simulink model "run_2022"  (R2022b)
settings: Solver=VariableStepAuto  StartTime=t_i  StopTime=2  MaxStep=s_max  RelTol=1e-3
InitFcn:
  | data;
  | init;
values from neighbouring files (symbols this model uses):
  h_ej = 0.15    [data.m]
  phi_0 = atan(-(r_ej*h_0)/(h_ej^2*sqrt(1-h_0^2/h_ej^2)))    [init.m]
  r_0 = sqrt((r_ej^2)*(1-h_0^2/h_ej^2))    [init.m]
  r_ej = 0.0821    [data.m]
  T_d = 1e-20    [data.m]
  x_ej = -0.05    [data.m]
  y_ej = 0.06    [data.m]
  z_ej = -0.03    [data.m]
undefined symbols (not defined in the file or in its folder): Glenohumeral_F0M, Glenohumeral_l0, Scapulothoracic_F0M, Scapulothoracic_l0, X, Y, Z
libraries: sm_lib x148, nesl_utility x62
(part 2 of 4)

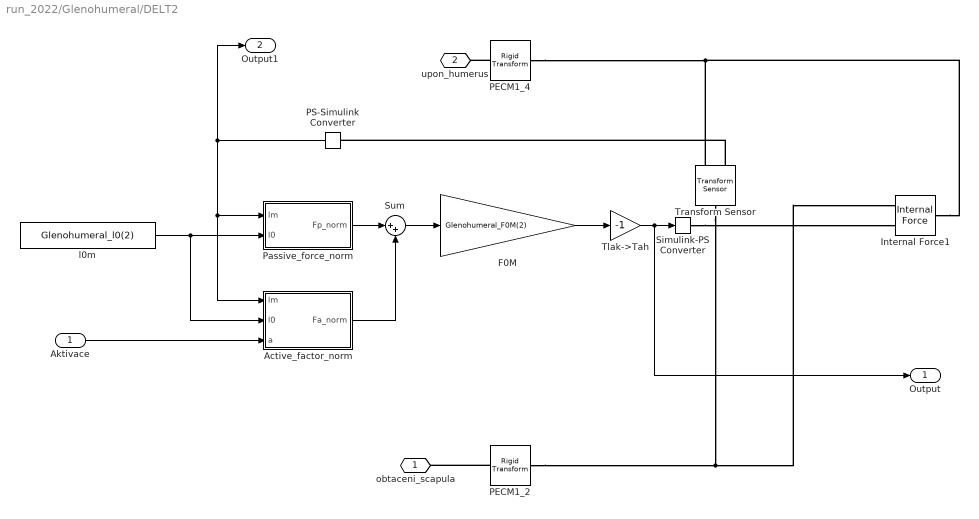
== system run_2022/Glenohumeral/DELT2 ==
  Aktivace : Inport
  Active_factor_norm : MATLAB Function  TreatAsAtomicUnit=on
  F0M : Gain  Gain=Glenohumeral_F0M(2)
  Internal Force1 : sm_lib/Forces and Torques/Internal Force
  PECM1_2 : sm_lib/Frames and Transforms/Rigid Transform  TranslationMethod=Cartesian  TranslationStandardOffset=0  TranslationStandardOffsetUnits=m  TranslationStandardAxis=+Z  TranslationCartesianOffset=[-0.028 -0.005 0.018]  TranslationCartesianOffsetUnits=m  TranslationROffset=0  TranslationROffsetUnits=m  TranslationZOffset=0  TranslationZOffsetUnits=m  TranslationThetaOffset=0  TranslationThetaOffsetUnits=deg  RotationMethod=None  RotationAngleUnits=deg  RotationStandardAxis=+Z  RotationAngle=0.0  RotationArbitraryAxis=[0 0 1]  FollAlignAxisA=+X  BaseAlignAxisA=+Y  FollAlignAxisB=+Y  BaseAlignAxisB=+Z  RotationSequenceAxes=FollowerAxes  RotationSequence=XYX  RotationSequenceAngles=[0 0 0]  RotationSequenceAnglesUnits=deg  RotationMatrix=[1 0 0; 0 1 0; 0 0 1]  Quaternion=[1 0 0 0]
  PECM1_4 : sm_lib/Frames and Transforms/Rigid Transform  TranslationMethod=Cartesian  TranslationStandardOffset=0  TranslationStandardOffsetUnits=m  TranslationStandardAxis=+Z  TranslationCartesianOffset=[-0.004 -0.058 0.028]  TranslationCartesianOffsetUnits=m  TranslationROffset=0  TranslationROffsetUnits=m  TranslationZOffset=0  TranslationZOffsetUnits=m  TranslationThetaOffset=0  TranslationThetaOffsetUnits=deg  RotationMethod=StandardAxis  RotationAngleUnits=deg  RotationStandardAxis=+Y  RotationAngle=90  RotationArbitraryAxis=[0 0 1]  FollAlignAxisA=+X  BaseAlignAxisA=+Y  FollAlignAxisB=+Y  BaseAlignAxisB=+Z  RotationSequenceAxes=FollowerAxes  RotationSequence=XYX  RotationSequenceAngles=[0 0 0]  RotationSequenceAnglesUnits=deg  RotationMatrix=[1 0 0; 0 1 0; 0 0 1]  Quaternion=[1 0 0 0]
  PS-Simulink Converter : nesl_utility/PS-Simulink Converter  PhysicalDomain=network_engine_domain  SubClassName=ps_output  LeftPortType=input  RightPortType=output  PseudoPeriodic=off  Frequencies=[]  VectorFormat=inherit  Unit=inherit  AffineConversion=off
  Passive_force_norm : MATLAB Function  TreatAsAtomicUnit=on
  Simulink-PS Converter : nesl_utility/Simulink-PS Converter  PhysicalDomain=network_engine_domain  SubClassName=ps_input  LeftPortType=input  RightPortType=output  PseudoPeriodic=off  Frequencies=[]  NoiseDistribution=none  NoiseParameters=[]  Unit=1  AffineConversion=off  FilteringAndDerivatives=provide  SimscapeFilterOrder=1  InputFilterTimeConstant=0.001  UdotUserProvided=0
  Sum : Sum  Inputs=|++
  Tlak->Tah : Gain  Gain=-1
  Transform Sensor : sm_lib/Frames and Transforms/Transform Sensor  MeasurementFrame=World  RotationSequence=XYX  SenseAngle=off  SenseAxis=off  SenseQ=off  SenseR=off  SenseRotationSequence=off  SenseOmegaX=off  SenseOmegaY=off  SenseOmegaZ=off  SenseQDot=off  SenseRDot=off  SenseRotationSequenceDot=off  SenseAlphaX=off  SenseAlphaY=off  SenseAlphaZ=off  SenseQDDot=off  SenseRDDot=off  SenseX=off  SenseY=off  SenseZ=off  SenseRad=off  SenseAzim=off  SenseDist=on  SenseInc=off  SenseXDot=off  SenseYDot=off  SenseZDot=off  SenseRadDot=off  SenseAzimDot=off  SenseDistDot=off  SenseIncDot=off  SenseXDDot=off  SenseYDDot=off  SenseZDDot=off  SenseRadDDot=off  SenseAzimDDot=off  SenseDistDDot=off  SenseIncDDot=off
  l0m : Constant  Value=Glenohumeral_l0(2)
  obtaceni_scapula : PMIOPort  Side=Left
  upon_humerus : PMIOPort  Port=2  Side=Left
  Output : Outport
  Output1 : Outport  Port=2
  wires:
  Passive_force_norm/1(Fp_norm) -> Sum/1
  F0M/1 -> Tlak->Tah/1
  Sum/1 -> F0M/1
  Active_factor_norm/1(Fa_norm) -> Sum/2
  Tlak->Tah/1 -> Output/1, Simulink-PS Converter/1
  PS-Simulink Converter/1 -> Output1/1, Active_factor_norm/1(lm), Passive_force_norm/1(lm)
  l0m/1 -> Active_factor_norm/2(l0), Passive_force_norm/2(l0)
  Aktivace/1 -> Active_factor_norm/3(a)
  connections:
  Transform Sensor/LConn1 -- PECM1_2/RConn1 -- Internal Force1/LConn1
  Transform Sensor/RConn1 -- PECM1_4/RConn1 -- Internal Force1/RConn1
  PECM1_2/LConn1 -- obtaceni_scapula/RConn1
  PECM1_4/LConn1 -- upon_humerus/RConn1
  Simulink-PS Converter/RConn1 -- Internal Force1/LConn2
  Transform Sensor/RConn2 -- PS-Simulink Converter/LConn1

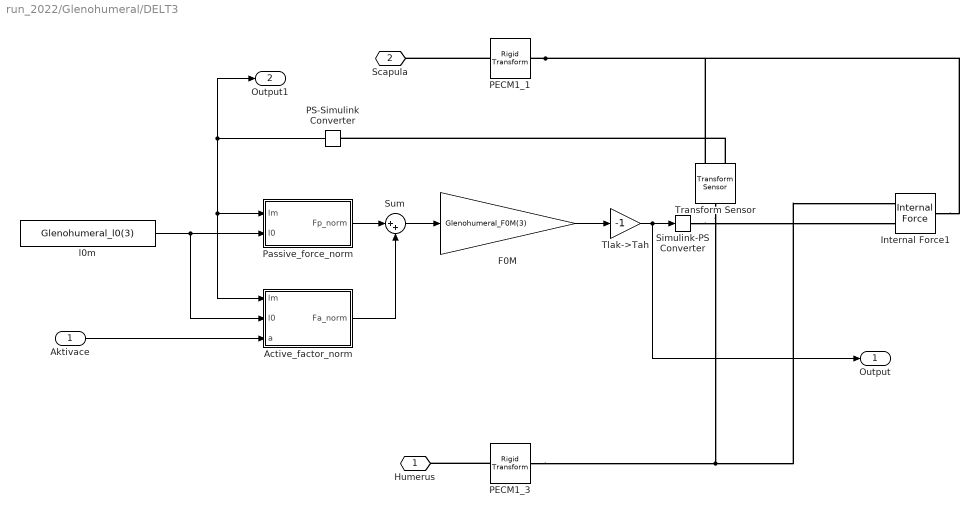
== system run_2022/Glenohumeral/DELT3 ==
  Aktivace : Inport
  Active_factor_norm : MATLAB Function  TreatAsAtomicUnit=on
  F0M : Gain  Gain=Glenohumeral_F0M(3)
  Internal Force1 : sm_lib/Forces and Torques/Internal Force
  PECM1_1 : sm_lib/Frames and Transforms/Rigid Transform  TranslationMethod=Cartesian  TranslationStandardOffset=0  TranslationStandardOffsetUnits=m  TranslationStandardAxis=+Z  TranslationCartesianOffset=[-0.072 -0.024 0.006]  TranslationCartesianOffsetUnits=m  TranslationROffset=0  TranslationROffsetUnits=m  TranslationZOffset=0  TranslationZOffsetUnits=m  TranslationThetaOffset=0  TranslationThetaOffsetUnits=deg  RotationMethod=None  RotationAngleUnits=deg  RotationStandardAxis=+Z  RotationAngle=0.0  RotationArbitraryAxis=[0 0 1]  FollAlignAxisA=+X  BaseAlignAxisA=+Y  FollAlignAxisB=+Y  BaseAlignAxisB=+Z  RotationSequenceAxes=FollowerAxes  RotationSequence=XYX  RotationSequenceAngles=[0 0 0]  RotationSequenceAnglesUnits=deg  RotationMatrix=[1 0 0; 0 1 0; 0 0 1]  Quaternion=[1 0 0 0]
  PECM1_3 : sm_lib/Frames and Transforms/Rigid Transform  TranslationMethod=Cartesian  TranslationStandardOffset=0  TranslationStandardOffsetUnits=m  TranslationStandardAxis=+Z  TranslationCartesianOffset=[-0.019 -0.05 0.006]  TranslationCartesianOffsetUnits=m  TranslationROffset=0  TranslationROffsetUnits=m  TranslationZOffset=0  TranslationZOffsetUnits=m  TranslationThetaOffset=0  TranslationThetaOffsetUnits=deg  RotationMethod=StandardAxis  RotationAngleUnits=deg  RotationStandardAxis=+Y  RotationAngle=90  RotationArbitraryAxis=[0 0 1]  FollAlignAxisA=+X  BaseAlignAxisA=+Y  FollAlignAxisB=+Y  BaseAlignAxisB=+Z  RotationSequenceAxes=FollowerAxes  RotationSequence=XYX  RotationSequenceAngles=[0 0 0]  RotationSequenceAnglesUnits=deg  RotationMatrix=[1 0 0; 0 1 0; 0 0 1]  Quaternion=[1 0 0 0]
  PS-Simulink Converter : nesl_utility/PS-Simulink Converter  PhysicalDomain=network_engine_domain  SubClassName=ps_output  LeftPortType=input  RightPortType=output  PseudoPeriodic=off  Frequencies=[]  VectorFormat=inherit  Unit=inherit  AffineConversion=off
  Passive_force_norm : MATLAB Function  TreatAsAtomicUnit=on
  Simulink-PS Converter : nesl_utility/Simulink-PS Converter  PhysicalDomain=network_engine_domain  SubClassName=ps_input  LeftPortType=input  RightPortType=output  PseudoPeriodic=off  Frequencies=[]  NoiseDistribution=none  NoiseParameters=[]  Unit=1  AffineConversion=off  FilteringAndDerivatives=provide  SimscapeFilterOrder=1  InputFilterTimeConstant=0.001  UdotUserProvided=0
  Sum : Sum  Inputs=|++
  Tlak->Tah : Gain  Gain=-1
  Transform Sensor : sm_lib/Frames and Transforms/Transform Sensor  MeasurementFrame=World  RotationSequence=XYX  SenseAngle=off  SenseAxis=off  SenseQ=off  SenseR=off  SenseRotationSequence=off  SenseOmegaX=off  SenseOmegaY=off  SenseOmegaZ=off  SenseQDot=off  SenseRDot=off  SenseRotationSequenceDot=off  SenseAlphaX=off  SenseAlphaY=off  SenseAlphaZ=off  SenseQDDot=off  SenseRDDot=off  SenseX=off  SenseY=off  SenseZ=off  SenseRad=off  SenseAzim=off  SenseDist=on  SenseInc=off  SenseXDot=off  SenseYDot=off  SenseZDot=off  SenseRadDot=off  SenseAzimDot=off  SenseDistDot=off  SenseIncDot=off  SenseXDDot=off  SenseYDDot=off  SenseZDDot=off  SenseRadDDot=off  SenseAzimDDot=off  SenseDistDDot=off  SenseIncDDot=off
  l0m : Constant  Value=Glenohumeral_l0(3)
  Humerus : PMIOPort  Side=Left
  Scapula : PMIOPort  Port=2  Side=Left
  Output : Outport
  Output1 : Outport  Port=2
  wires:
  l0m/1 -> Active_factor_norm/2(l0), Passive_force_norm/2(l0)
  Tlak->Tah/1 -> Output/1, Simulink-PS Converter/1
  PS-Simulink Converter/1 -> Output1/1, Active_factor_norm/1(lm), Passive_force_norm/1(lm)
  Active_factor_norm/1(Fa_norm) -> Sum/2
  Sum/1 -> F0M/1
  Passive_force_norm/1(Fp_norm) -> Sum/1
  F0M/1 -> Tlak->Tah/1
  Aktivace/1 -> Active_factor_norm/3(a)
  connections:
  PECM1_1/RConn1 -- Internal Force1/RConn1 -- Transform Sensor/RConn1
  PECM1_3/RConn1 -- Internal Force1/LConn1 -- Transform Sensor/LConn1
  Transform Sensor/RConn2 -- PS-Simulink Converter/LConn1
  Simulink-PS Converter/RConn1 -- Internal Force1/LConn2
  PECM1_3/LConn1 -- Humerus/RConn1
  PECM1_1/LConn1 -- Scapula/RConn1

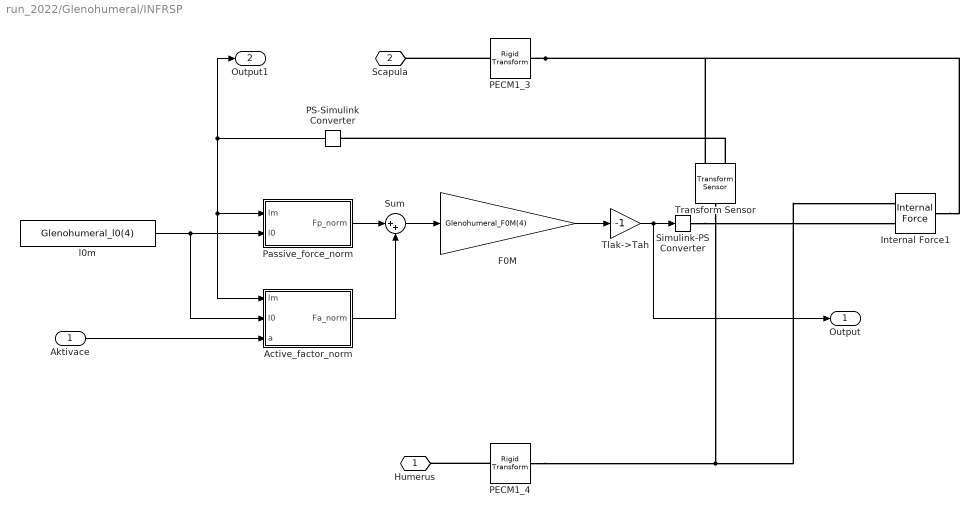
== system run_2022/Glenohumeral/INFRSP ==
  Aktivace : Inport
  Active_factor_norm : MATLAB Function  TreatAsAtomicUnit=on
  F0M : Gain  Gain=Glenohumeral_F0M(4)
  Internal Force1 : sm_lib/Forces and Torques/Internal Force
  PECM1_3 : sm_lib/Frames and Transforms/Rigid Transform  TranslationMethod=Cartesian  TranslationStandardOffset=0  TranslationStandardOffsetUnits=m  TranslationStandardAxis=+Z  TranslationCartesianOffset=[-0.043 -0.048 -0.022]  TranslationCartesianOffsetUnits=m  TranslationROffset=0  TranslationROffsetUnits=m  TranslationZOffset=0  TranslationZOffsetUnits=m  TranslationThetaOffset=0  TranslationThetaOffsetUnits=deg  RotationMethod=None  RotationAngleUnits=deg  RotationStandardAxis=+Z  RotationAngle=0.0  RotationArbitraryAxis=[0 0 1]  FollAlignAxisA=+X  BaseAlignAxisA=+Y  FollAlignAxisB=+Y  BaseAlignAxisB=+Z  RotationSequenceAxes=FollowerAxes  RotationSequence=XYX  RotationSequenceAngles=[0 0 0]  RotationSequenceAnglesUnits=deg  RotationMatrix=[1 0 0; 0 1 0; 0 0 1]  Quaternion=[1 0 0 0]
  PECM1_4 : sm_lib/Frames and Transforms/Rigid Transform  TranslationMethod=Cartesian  TranslationStandardOffset=0  TranslationStandardOffsetUnits=m  TranslationStandardAxis=+Z  TranslationCartesianOffset=[-0.005 0.008 0.026]  TranslationCartesianOffsetUnits=m  TranslationROffset=0  TranslationROffsetUnits=m  TranslationZOffset=0  TranslationZOffsetUnits=m  TranslationThetaOffset=0  TranslationThetaOffsetUnits=deg  RotationMethod=StandardAxis  RotationAngleUnits=deg  RotationStandardAxis=+Y  RotationAngle=90  RotationArbitraryAxis=[0 0 1]  FollAlignAxisA=+X  BaseAlignAxisA=+Y  FollAlignAxisB=+Y  BaseAlignAxisB=+Z  RotationSequenceAxes=FollowerAxes  RotationSequence=XYX  RotationSequenceAngles=[0 0 0]  RotationSequenceAnglesUnits=deg  RotationMatrix=[1 0 0; 0 1 0; 0 0 1]  Quaternion=[1 0 0 0]
  PS-Simulink Converter : nesl_utility/PS-Simulink Converter  PhysicalDomain=network_engine_domain  SubClassName=ps_output  LeftPortType=input  RightPortType=output  PseudoPeriodic=off  Frequencies=[]  VectorFormat=inherit  Unit=inherit  AffineConversion=off
  Passive_force_norm : MATLAB Function  TreatAsAtomicUnit=on
  Simulink-PS Converter : nesl_utility/Simulink-PS Converter  PhysicalDomain=network_engine_domain  SubClassName=ps_input  LeftPortType=input  RightPortType=output  PseudoPeriodic=off  Frequencies=[]  NoiseDistribution=none  NoiseParameters=[]  Unit=1  AffineConversion=off  FilteringAndDerivatives=provide  SimscapeFilterOrder=1  InputFilterTimeConstant=0.001  UdotUserProvided=0
  Sum : Sum  Inputs=|++
  Tlak->Tah : Gain  Gain=-1
  Transform Sensor : sm_lib/Frames and Transforms/Transform Sensor  MeasurementFrame=World  RotationSequence=XYX  SenseAngle=off  SenseAxis=off  SenseQ=off  SenseR=off  SenseRotationSequence=off  SenseOmegaX=off  SenseOmegaY=off  SenseOmegaZ=off  SenseQDot=off  SenseRDot=off  SenseRotationSequenceDot=off  SenseAlphaX=off  SenseAlphaY=off  SenseAlphaZ=off  SenseQDDot=off  SenseRDDot=off  SenseX=off  SenseY=off  SenseZ=off  SenseRad=off  SenseAzim=off  SenseDist=on  SenseInc=off  SenseXDot=off  SenseYDot=off  SenseZDot=off  SenseRadDot=off  SenseAzimDot=off  SenseDistDot=off  SenseIncDot=off  SenseXDDot=off  SenseYDDot=off  SenseZDDot=off  SenseRadDDot=off  SenseAzimDDot=off  SenseDistDDot=off  SenseIncDDot=off
  l0m : Constant  Value=Glenohumeral_l0(4)
  Humerus : PMIOPort  Side=Left
  Scapula : PMIOPort  Port=2  Side=Left
  Output : Outport
  Output1 : Outport  Port=2
  wires:
  PS-Simulink Converter/1 -> Output1/1, Active_factor_norm/1(lm), Passive_force_norm/1(lm)
  l0m/1 -> Active_factor_norm/2(l0), Passive_force_norm/2(l0)
  Tlak->Tah/1 -> Output/1, Simulink-PS Converter/1
  Sum/1 -> F0M/1
  F0M/1 -> Tlak->Tah/1
  Aktivace/1 -> Active_factor_norm/3(a)
  Passive_force_norm/1(Fp_norm) -> Sum/1
  Active_factor_norm/1(Fa_norm) -> Sum/2
  connections:
  PECM1_4/RConn1 -- Internal Force1/LConn1 -- Transform Sensor/LConn1
  PECM1_3/RConn1 -- Internal Force1/RConn1 -- Transform Sensor/RConn1
  PECM1_3/LConn1 -- Scapula/RConn1
  Simulink-PS Converter/RConn1 -- Internal Force1/LConn2
  PECM1_4/LConn1 -- Humerus/RConn1
  Transform Sensor/RConn2 -- PS-Simulink Converter/LConn1

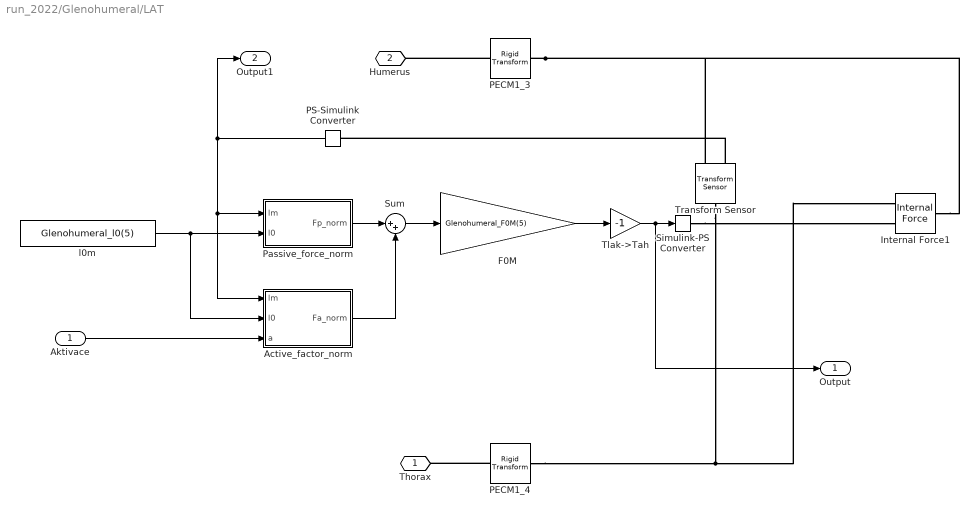
== system run_2022/Glenohumeral/LAT ==
  Aktivace : Inport
  Active_factor_norm : MATLAB Function  TreatAsAtomicUnit=on
  F0M : Gain  Gain=Glenohumeral_F0M(5)
  Internal Force1 : sm_lib/Forces and Torques/Internal Force
  PECM1_3 : sm_lib/Frames and Transforms/Rigid Transform  TranslationMethod=Cartesian  TranslationStandardOffset=0  TranslationStandardOffsetUnits=m  TranslationStandardAxis=+Z  TranslationCartesianOffset=[0.002 -0.019 -0.021]  TranslationCartesianOffsetUnits=m  TranslationROffset=0  TranslationROffsetUnits=m  TranslationZOffset=0  TranslationZOffsetUnits=m  TranslationThetaOffset=0  TranslationThetaOffsetUnits=deg  RotationMethod=None  RotationAngleUnits=deg  RotationStandardAxis=+Z  RotationAngle=0.0  RotationArbitraryAxis=[0 0 1]  FollAlignAxisA=+X  BaseAlignAxisA=+Y  FollAlignAxisB=+Y  BaseAlignAxisB=+Z  RotationSequenceAxes=FollowerAxes  RotationSequence=XYX  RotationSequenceAngles=[0 0 0]  RotationSequenceAnglesUnits=deg  RotationMatrix=[1 0 0; 0 1 0; 0 0 1]  Quaternion=[1 0 0 0]
  PECM1_4 : sm_lib/Frames and Transforms/Rigid Transform  TranslationMethod=Cartesian  TranslationStandardOffset=0  TranslationStandardOffsetUnits=m  TranslationStandardAxis=+Z  TranslationCartesianOffset=[-0.095 -0.161 0.001]  TranslationCartesianOffsetUnits=m  TranslationROffset=0  TranslationROffsetUnits=m  TranslationZOffset=0  TranslationZOffsetUnits=m  TranslationThetaOffset=0  TranslationThetaOffsetUnits=deg  RotationMethod=StandardAxis  RotationAngleUnits=deg  RotationStandardAxis=+Y  RotationAngle=90  RotationArbitraryAxis=[0 0 1]  FollAlignAxisA=+X  BaseAlignAxisA=+Y  FollAlignAxisB=+Y  BaseAlignAxisB=+Z  RotationSequenceAxes=FollowerAxes  RotationSequence=XYX  RotationSequenceAngles=[0 0 0]  RotationSequenceAnglesUnits=deg  RotationMatrix=[1 0 0; 0 1 0; 0 0 1]  Quaternion=[1 0 0 0]
  PS-Simulink Converter : nesl_utility/PS-Simulink Converter  PhysicalDomain=network_engine_domain  SubClassName=ps_output  LeftPortType=input  RightPortType=output  PseudoPeriodic=off  Frequencies=[]  VectorFormat=inherit  Unit=inherit  AffineConversion=off
  Passive_force_norm : MATLAB Function  TreatAsAtomicUnit=on
  Simulink-PS Converter : nesl_utility/Simulink-PS Converter  PhysicalDomain=network_engine_domain  SubClassName=ps_input  LeftPortType=input  RightPortType=output  PseudoPeriodic=off  Frequencies=[]  NoiseDistribution=none  NoiseParameters=[]  Unit=1  AffineConversion=off  FilteringAndDerivatives=provide  SimscapeFilterOrder=1  InputFilterTimeConstant=0.001  UdotUserProvided=0
  Sum : Sum  Inputs=|++
  Tlak->Tah : Gain  Gain=-1
  Transform Sensor : sm_lib/Frames and Transforms/Transform Sensor  MeasurementFrame=World  RotationSequence=XYX  SenseAngle=off  SenseAxis=off  SenseQ=off  SenseR=off  SenseRotationSequence=off  SenseOmegaX=off  SenseOmegaY=off  SenseOmegaZ=off  SenseQDot=off  SenseRDot=off  SenseRotationSequenceDot=off  SenseAlphaX=off  SenseAlphaY=off  SenseAlphaZ=off  SenseQDDot=off  SenseRDDot=off  SenseX=off  SenseY=off  SenseZ=off  SenseRad=off  SenseAzim=off  SenseDist=on  SenseInc=off  SenseXDot=off  SenseYDot=off  SenseZDot=off  SenseRadDot=off  SenseAzimDot=off  SenseDistDot=off  SenseIncDot=off  SenseXDDot=off  SenseYDDot=off  SenseZDDot=off  SenseRadDDot=off  SenseAzimDDot=off  SenseDistDDot=off  SenseIncDDot=off
  l0m : Constant  Value=Glenohumeral_l0(5)
  Thorax : PMIOPort  Side=Left
  Humerus : PMIOPort  Port=2  Side=Left
  Output : Outport
  Output1 : Outport  Port=2
  wires:
  Active_factor_norm/1(Fa_norm) -> Sum/2
  Passive_force_norm/1(Fp_norm) -> Sum/1
  Tlak->Tah/1 -> Output/1, Simulink-PS Converter/1
  Aktivace/1 -> Active_factor_norm/3(a)
  PS-Simulink Converter/1 -> Output1/1, Active_factor_norm/1(lm), Passive_force_norm/1(lm)
  F0M/1 -> Tlak->Tah/1
  l0m/1 -> Active_factor_norm/2(l0), Passive_force_norm/2(l0)
  Sum/1 -> F0M/1
  connections:
  PECM1_4/RConn1 -- Internal Force1/LConn1 -- Transform Sensor/LConn1
  PECM1_3/RConn1 -- Internal Force1/RConn1 -- Transform Sensor/RConn1
  PECM1_3/LConn1 -- Humerus/RConn1
  PECM1_4/LConn1 -- Thorax/RConn1
  Simulink-PS Converter/RConn1 -- Internal Force1/LConn2
  Transform Sensor/RConn2 -- PS-Simulink Converter/LConn1

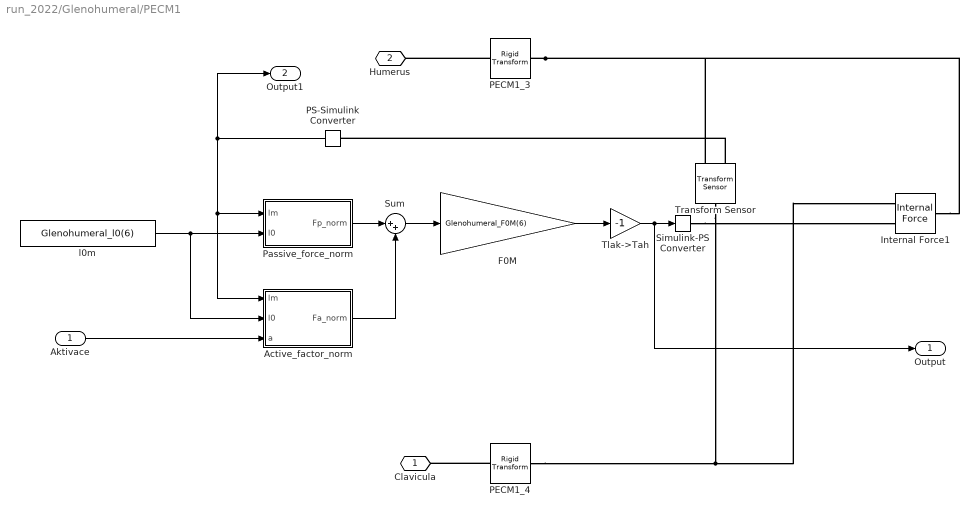
== system run_2022/Glenohumeral/PECM1 ==
  Aktivace : Inport
  Active_factor_norm : MATLAB Function  TreatAsAtomicUnit=on
  F0M : Gain  Gain=Glenohumeral_F0M(6)
  Internal Force1 : sm_lib/Forces and Torques/Internal Force
  PECM1_3 : sm_lib/Frames and Transforms/Rigid Transform  TranslationMethod=Cartesian  TranslationStandardOffset=0  TranslationStandardOffsetUnits=m  TranslationStandardAxis=+Z  TranslationCartesianOffset=[0.016 -0.04 0.005]  TranslationCartesianOffsetUnits=m  TranslationROffset=0  TranslationROffsetUnits=m  TranslationZOffset=0  TranslationZOffsetUnits=m  TranslationThetaOffset=0  TranslationThetaOffsetUnits=deg  RotationMethod=None  RotationAngleUnits=deg  RotationStandardAxis=+Z  RotationAngle=0.0  RotationArbitraryAxis=[0 0 1]  FollAlignAxisA=+X  BaseAlignAxisA=+Y  FollAlignAxisB=+Y  BaseAlignAxisB=+Z  RotationSequenceAxes=FollowerAxes  RotationSequence=XYX  RotationSequenceAngles=[0 0 0]  RotationSequenceAnglesUnits=deg  RotationMatrix=[1 0 0; 0 1 0; 0 0 1]  Quaternion=[1 0 0 0]
  PECM1_4 : sm_lib/Frames and Transforms/Rigid Transform  TranslationMethod=Cartesian  TranslationStandardOffset=0  TranslationStandardOffsetUnits=m  TranslationStandardAxis=+Z  TranslationCartesianOffset=[0 0.006 0.059]  TranslationCartesianOffsetUnits=m  TranslationROffset=0  TranslationROffsetUnits=m  TranslationZOffset=0  TranslationZOffsetUnits=m  TranslationThetaOffset=0  TranslationThetaOffsetUnits=deg  RotationMethod=StandardAxis  RotationAngleUnits=deg  RotationStandardAxis=+Y  RotationAngle=90  RotationArbitraryAxis=[0 0 1]  FollAlignAxisA=+X  BaseAlignAxisA=+Y  FollAlignAxisB=+Y  BaseAlignAxisB=+Z  RotationSequenceAxes=FollowerAxes  RotationSequence=XYX  RotationSequenceAngles=[0 0 0]  RotationSequenceAnglesUnits=deg  RotationMatrix=[1 0 0; 0 1 0; 0 0 1]  Quaternion=[1 0 0 0]
  PS-Simulink Converter : nesl_utility/PS-Simulink Converter  PhysicalDomain=network_engine_domain  SubClassName=ps_output  LeftPortType=input  RightPortType=output  PseudoPeriodic=off  Frequencies=[]  VectorFormat=inherit  Unit=inherit  AffineConversion=off
  Passive_force_norm : MATLAB Function  TreatAsAtomicUnit=on
  Simulink-PS Converter : nesl_utility/Simulink-PS Converter  PhysicalDomain=network_engine_domain  SubClassName=ps_input  LeftPortType=input  RightPortType=output  PseudoPeriodic=off  Frequencies=[]  NoiseDistribution=none  NoiseParameters=[]  Unit=1  AffineConversion=off  FilteringAndDerivatives=provide  SimscapeFilterOrder=1  InputFilterTimeConstant=0.001  UdotUserProvided=0
  Sum : Sum  Inputs=|++
  Tlak->Tah : Gain  Gain=-1
  Transform Sensor : sm_lib/Frames and Transforms/Transform Sensor  MeasurementFrame=World  RotationSequence=XYX  SenseAngle=off  SenseAxis=off  SenseQ=off  SenseR=off  SenseRotationSequence=off  SenseOmegaX=off  SenseOmegaY=off  SenseOmegaZ=off  SenseQDot=off  SenseRDot=off  SenseRotationSequenceDot=off  SenseAlphaX=off  SenseAlphaY=off  SenseAlphaZ=off  SenseQDDot=off  SenseRDDot=off  SenseX=off  SenseY=off  SenseZ=off  SenseRad=off  SenseAzim=off  SenseDist=on  SenseInc=off  SenseXDot=off  SenseYDot=off  SenseZDot=off  SenseRadDot=off  SenseAzimDot=off  SenseDistDot=off  SenseIncDot=off  SenseXDDot=off  SenseYDDot=off  SenseZDDot=off  SenseRadDDot=off  SenseAzimDDot=off  SenseDistDDot=off  SenseIncDDot=off
  l0m : Constant  Value=Glenohumeral_l0(6)
  Clavicula : PMIOPort  Side=Left
  Humerus : PMIOPort  Port=2  Side=Left
  Output : Outport
  Output1 : Outport  Port=2
  wires:
  Tlak->Tah/1 -> Output/1, Simulink-PS Converter/1
  l0m/1 -> Active_factor_norm/2(l0), Passive_force_norm/2(l0)
  Passive_force_norm/1(Fp_norm) -> Sum/1
  F0M/1 -> Tlak->Tah/1
  Aktivace/1 -> Active_factor_norm/3(a)
  Sum/1 -> F0M/1
  Active_factor_norm/1(Fa_norm) -> Sum/2
  PS-Simulink Converter/1 -> Output1/1, Active_factor_norm/1(lm), Passive_force_norm/1(lm)
  connections:
  PECM1_3/RConn1 -- Internal Force1/RConn1 -- Transform Sensor/RConn1
  PECM1_4/RConn1 -- Internal Force1/LConn1 -- Transform Sensor/LConn1
  PECM1_3/LConn1 -- Humerus/RConn1
  PECM1_4/LConn1 -- Clavicula/RConn1
  Transform Sensor/RConn2 -- PS-Simulink Converter/LConn1
  Simulink-PS Converter/RConn1 -- Internal Force1/LConn2

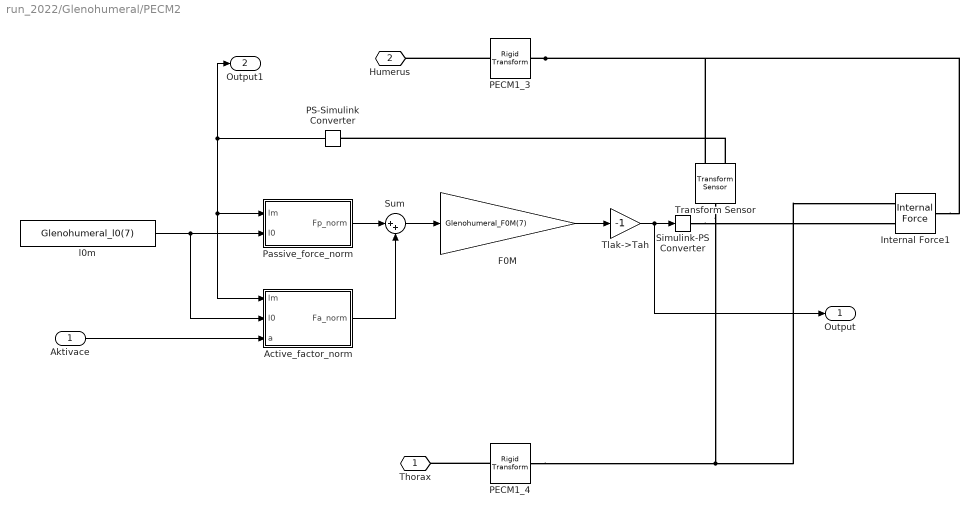
== system run_2022/Glenohumeral/PECM2 ==
  Aktivace : Inport
  Active_factor_norm : MATLAB Function  TreatAsAtomicUnit=on
  F0M : Gain  Gain=Glenohumeral_F0M(7)
  Internal Force1 : sm_lib/Forces and Torques/Internal Force
  PECM1_3 : sm_lib/Frames and Transforms/Rigid Transform  TranslationMethod=Cartesian  TranslationStandardOffset=0  TranslationStandardOffsetUnits=m  TranslationStandardAxis=+Z  TranslationCartesianOffset=[0.016 -0.035 0.005]  TranslationCartesianOffsetUnits=m  TranslationROffset=0  TranslationROffsetUnits=m  TranslationZOffset=0  TranslationZOffsetUnits=m  TranslationThetaOffset=0  TranslationThetaOffsetUnits=deg  RotationMethod=None  RotationAngleUnits=deg  RotationStandardAxis=+Z  RotationAngle=0.0  RotationArbitraryAxis=[0 0 1]  FollAlignAxisA=+X  BaseAlignAxisA=+Y  FollAlignAxisB=+Y  BaseAlignAxisB=+Z  RotationSequenceAxes=FollowerAxes  RotationSequence=XYX  RotationSequenceAngles=[0 0 0]  RotationSequenceAnglesUnits=deg  RotationMatrix=[1 0 0; 0 1 0; 0 0 1]  Quaternion=[1 0 0 0]
  PECM1_4 : sm_lib/Frames and Transforms/Rigid Transform  TranslationMethod=Cartesian  TranslationStandardOffset=0  TranslationStandardOffsetUnits=m  TranslationStandardAxis=+Z  TranslationCartesianOffset=[0.042 -0.043 0.081]  TranslationCartesianOffsetUnits=m  TranslationROffset=0  TranslationROffsetUnits=m  TranslationZOffset=0  TranslationZOffsetUnits=m  TranslationThetaOffset=0  TranslationThetaOffsetUnits=deg  RotationMethod=StandardAxis  RotationAngleUnits=deg  RotationStandardAxis=+Y  RotationAngle=90  RotationArbitraryAxis=[0 0 1]  FollAlignAxisA=+X  BaseAlignAxisA=+Y  FollAlignAxisB=+Y  BaseAlignAxisB=+Z  RotationSequenceAxes=FollowerAxes  RotationSequence=XYX  RotationSequenceAngles=[0 0 0]  RotationSequenceAnglesUnits=deg  RotationMatrix=[1 0 0; 0 1 0; 0 0 1]  Quaternion=[1 0 0 0]
  PS-Simulink Converter : nesl_utility/PS-Simulink Converter  PhysicalDomain=network_engine_domain  SubClassName=ps_output  LeftPortType=input  RightPortType=output  PseudoPeriodic=off  Frequencies=[]  VectorFormat=inherit  Unit=inherit  AffineConversion=off
  Passive_force_norm : MATLAB Function  TreatAsAtomicUnit=on
  Simulink-PS Converter : nesl_utility/Simulink-PS Converter  PhysicalDomain=network_engine_domain  SubClassName=ps_input  LeftPortType=input  RightPortType=output  PseudoPeriodic=off  Frequencies=[]  NoiseDistribution=none  NoiseParameters=[]  Unit=1  AffineConversion=off  FilteringAndDerivatives=provide  SimscapeFilterOrder=1  InputFilterTimeConstant=0.001  UdotUserProvided=0
  Sum : Sum  Inputs=|++
  Tlak->Tah : Gain  Gain=-1
  Transform Sensor : sm_lib/Frames and Transforms/Transform Sensor  MeasurementFrame=World  RotationSequence=XYX  SenseAngle=off  SenseAxis=off  SenseQ=off  SenseR=off  SenseRotationSequence=off  SenseOmegaX=off  SenseOmegaY=off  SenseOmegaZ=off  SenseQDot=off  SenseRDot=off  SenseRotationSequenceDot=off  SenseAlphaX=off  SenseAlphaY=off  SenseAlphaZ=off  SenseQDDot=off  SenseRDDot=off  SenseX=off  SenseY=off  SenseZ=off  SenseRad=off  SenseAzim=off  SenseDist=on  SenseInc=off  SenseXDot=off  SenseYDot=off  SenseZDot=off  SenseRadDot=off  SenseAzimDot=off  SenseDistDot=off  SenseIncDot=off  SenseXDDot=off  SenseYDDot=off  SenseZDDot=off  SenseRadDDot=off  SenseAzimDDot=off  SenseDistDDot=off  SenseIncDDot=off
  l0m : Constant  Value=Glenohumeral_l0(7)
  Thorax : PMIOPort  Side=Left
  Humerus : PMIOPort  Port=2  Side=Left
  Output : Outport
  Output1 : Outport  Port=2
  wires:
  l0m/1 -> Active_factor_norm/2(l0), Passive_force_norm/2(l0)
  Tlak->Tah/1 -> Output/1, Simulink-PS Converter/1
  PS-Simulink Converter/1 -> Output1/1, Active_factor_norm/1(lm), Passive_force_norm/1(lm)
  Aktivace/1 -> Active_factor_norm/3(a)
  Sum/1 -> F0M/1
  Active_factor_norm/1(Fa_norm) -> Sum/2
  Passive_force_norm/1(Fp_norm) -> Sum/1
  F0M/1 -> Tlak->Tah/1
  connections:
  PECM1_3/RConn1 -- Internal Force1/RConn1 -- Transform Sensor/RConn1
  PECM1_4/RConn1 -- Internal Force1/LConn1 -- Transform Sensor/LConn1
  PECM1_3/LConn1 -- Humerus/RConn1
  PECM1_4/LConn1 -- Thorax/RConn1
  Simulink-PS Converter/RConn1 -- Internal Force1/LConn2
  Transform Sensor/RConn2 -- PS-Simulink Converter/LConn1

== system run_2022/Glenohumeral/PECM3 ==
  Aktivace : Inport
  Active_factor_norm : MATLAB Function  TreatAsAtomicUnit=on
  F0M : Gain  Gain=Glenohumeral_F0M(8)
  Internal Force1 : sm_lib/Forces and Torques/Internal Force
  PECM1_3 : sm_lib/Frames and Transforms/Rigid Transform  TranslationMethod=Cartesian  TranslationStandardOffset=0  TranslationStandardOffsetUnits=m  TranslationStandardAxis=+Z  TranslationCartesianOffset=[0.016 -0.03 0.005]  TranslationCartesianOffsetUnits=m  TranslationROffset=0  TranslationROffsetUnits=m  TranslationZOffset=0  TranslationZOffsetUnits=m  TranslationThetaOffset=0  TranslationThetaOffsetUnits=deg  RotationMethod=None  RotationAngleUnits=deg  RotationStandardAxis=+Z  RotationAngle=0.0  RotationArbitraryAxis=[0 0 1]  FollAlignAxisA=+X  BaseAlignAxisA=+Y  FollAlignAxisB=+Y  BaseAlignAxisB=+Z  RotationSequenceAxes=FollowerAxes  RotationSequence=XYX  RotationSequenceAngles=[0 0 0]  RotationSequenceAnglesUnits=deg  RotationMatrix=[1 0 0; 0 1 0; 0 0 1]  Quaternion=[1 0 0 0]
  PECM1_4 : sm_lib/Frames and Transforms/Rigid Transform  TranslationMethod=Cartesian  TranslationStandardOffset=0  TranslationStandardOffsetUnits=m  TranslationStandardAxis=+Z  TranslationCartesianOffset=[0.043 -0.093 0.083]  TranslationCartesianOffsetUnits=m  TranslationROffset=0  TranslationROffsetUnits=m  TranslationZOffset=0  TranslationZOffsetUnits=m  TranslationThetaOffset=0  TranslationThetaOffsetUnits=deg  RotationMethod=StandardAxis  RotationAngleUnits=deg  RotationStandardAxis=+Y  RotationAngle=90  RotationArbitraryAxis=[0 0 1]  FollAlignAxisA=+X  BaseAlignAxisA=+Y  FollAlignAxisB=+Y  BaseAlignAxisB=+Z  RotationSequenceAxes=FollowerAxes  RotationSequence=XYX  RotationSequenceAngles=[0 0 0]  RotationSequenceAnglesUnits=deg  RotationMatrix=[1 0 0; 0 1 0; 0 0 1]  Quaternion=[1 0 0 0]
  PS-Simulink Converter : nesl_utility/PS-Simulink Converter  PhysicalDomain=network_engine_domain  SubClassName=ps_output  LeftPortType=input  RightPortType=output  PseudoPeriodic=off  Frequencies=[]  VectorFormat=inherit  Unit=inherit  AffineConversion=off
  Passive_force_norm : MATLAB Function  TreatAsAtomicUnit=on
  Simulink-PS Converter : nesl_utility/Simulink-PS Converter  PhysicalDomain=network_engine_domain  SubClassName=ps_input  LeftPortType=input  RightPortType=output  PseudoPeriodic=off  Frequencies=[]  NoiseDistribution=none  NoiseParameters=[]  Unit=1  AffineConversion=off  FilteringAndDerivatives=provide  SimscapeFilterOrder=1  InputFilterTimeConstant=0.001  UdotUserProvided=0
  Sum : Sum  Inputs=|++
  Tlak->Tah : Gain  Gain=-1
  Transform Sensor : sm_lib/Frames and Transforms/Transform Sensor  MeasurementFrame=World  RotationSequence=XYX  SenseAngle=off  SenseAxis=off  SenseQ=off  SenseR=off  SenseRotationSequence=off  SenseOmegaX=off  SenseOmegaY=off  SenseOmegaZ=off  SenseQDot=off  SenseRDot=off  SenseRotationSequenceDot=off  SenseAlphaX=off  SenseAlphaY=off  SenseAlphaZ=off  SenseQDDot=off  SenseRDDot=off  SenseX=off  SenseY=off  SenseZ=off  SenseRad=off  SenseAzim=off  SenseDist=on  SenseInc=off  SenseXDot=off  SenseYDot=off  SenseZDot=off  SenseRadDot=off  SenseAzimDot=off  SenseDistDot=off  SenseIncDot=off  SenseXDDot=off  SenseYDDot=off  SenseZDDot=off  SenseRadDDot=off  SenseAzimDDot=off  SenseDistDDot=off  SenseIncDDot=off
  l0m : Constant  Value=Glenohumeral_l0(8)
  Thorax : PMIOPort  Side=Left
  Humerus : PMIOPort  Port=2  Side=Left
  Output : Outport
  Output1 : Outport  Port=2
  wires:
  Aktivace/1 -> Active_factor_norm/3(a)
  F0M/1 -> Tlak->Tah/1
  Tlak->Tah/1 -> Output/1, Simulink-PS Converter/1
  Sum/1 -> F0M/1
  Active_factor_norm/1(Fa_norm) -> Sum/2
  Passive_force_norm/1(Fp_norm) -> Sum/1
  PS-Simulink Converter/1 -> Output1/1, Active_factor_norm/1(lm), Passive_force_norm/1(lm)
  l0m/1 -> Active_factor_norm/2(l0), Passive_force_norm/2(l0)
  connections:
  PECM1_4/RConn1 -- Internal Force1/LConn1 -- Transform Sensor/LConn1
  PECM1_3/RConn1 -- Internal Force1/RConn1 -- Transform Sensor/RConn1
  Simulink-PS Converter/RConn1 -- Internal Force1/LConn2
  PECM1_3/LConn1 -- Humerus/RConn1
  Transform Sensor/RConn2 -- PS-Simulink Converter/LConn1
  PECM1_4/LConn1 -- Thorax/RConn1

== system run_2022/Glenohumeral/SUBSC ==
  Aktivace : Inport
  Active_factor_norm : MATLAB Function  TreatAsAtomicUnit=on
  F0M : Gain  Gain=Glenohumeral_F0M(9)
  Internal Force1 : sm_lib/Forces and Torques/Internal Force
  PECM1_3 : sm_lib/Frames and Transforms/Rigid Transform  TranslationMethod=Cartesian  TranslationStandardOffset=0  TranslationStandardOffsetUnits=m  TranslationStandardAxis=+Z  TranslationCartesianOffset=[0.007 0.01 -0.023]  TranslationCartesianOffsetUnits=m  TranslationROffset=0  TranslationROffsetUnits=m  TranslationZOffset=0  TranslationZOffsetUnits=m  TranslationThetaOffset=0  TranslationThetaOffsetUnits=deg  RotationMethod=None  RotationAngleUnits=deg  RotationStandardAxis=+Z  RotationAngle=0.0  RotationArbitraryAxis=[0 0 1]  FollAlignAxisA=+X  BaseAlignAxisA=+Y  FollAlignAxisB=+Y  BaseAlignAxisB=+Z  RotationSequenceAxes=FollowerAxes  RotationSequence=XYX  RotationSequenceAngles=[0 0 0]  RotationSequenceAnglesUnits=deg  RotationMatrix=[1 0 0; 0 1 0; 0 0 1]  Quaternion=[1 0 0 0]
  PECM1_4 : sm_lib/Frames and Transforms/Rigid Transform  TranslationMethod=Cartesian  TranslationStandardOffset=0  TranslationStandardOffsetUnits=m  TranslationStandardAxis=+Z  TranslationCartesianOffset=[-0.039 -0.032 -0.033]  TranslationCartesianOffsetUnits=m  TranslationROffset=0  TranslationROffsetUnits=m  TranslationZOffset=0  TranslationZOffsetUnits=m  TranslationThetaOffset=0  TranslationThetaOffsetUnits=deg  RotationMethod=StandardAxis  RotationAngleUnits=deg  RotationStandardAxis=+Y  RotationAngle=90  RotationArbitraryAxis=[0 0 1]  FollAlignAxisA=+X  BaseAlignAxisA=+Y  FollAlignAxisB=+Y  BaseAlignAxisB=+Z  RotationSequenceAxes=FollowerAxes  RotationSequence=XYX  RotationSequenceAngles=[0 0 0]  RotationSequenceAnglesUnits=deg  RotationMatrix=[1 0 0; 0 1 0; 0 0 1]  Quaternion=[1 0 0 0]
  PS-Simulink Converter : nesl_utility/PS-Simulink Converter  PhysicalDomain=network_engine_domain  SubClassName=ps_output  LeftPortType=input  RightPortType=output  PseudoPeriodic=off  Frequencies=[]  VectorFormat=inherit  Unit=inherit  AffineConversion=off
  Passive_force_norm : MATLAB Function  TreatAsAtomicUnit=on
  Simulink-PS Converter : nesl_utility/Simulink-PS Converter  PhysicalDomain=network_engine_domain  SubClassName=ps_input  LeftPortType=input  RightPortType=output  PseudoPeriodic=off  Frequencies=[]  NoiseDistribution=none  NoiseParameters=[]  Unit=1  AffineConversion=off  FilteringAndDerivatives=provide  SimscapeFilterOrder=1  InputFilterTimeConstant=0.001  UdotUserProvided=0
  Sum : Sum  Inputs=|++
  Tlak->Tah : Gain  Gain=-1
  Transform Sensor : sm_lib/Frames and Transforms/Transform Sensor  MeasurementFrame=World  RotationSequence=XYX  SenseAngle=off  SenseAxis=off  SenseQ=off  SenseR=off  SenseRotationSequence=off  SenseOmegaX=off  SenseOmegaY=off  SenseOmegaZ=off  SenseQDot=off  SenseRDot=off  SenseRotationSequenceDot=off  SenseAlphaX=off  SenseAlphaY=off  SenseAlphaZ=off  SenseQDDot=off  SenseRDDot=off  SenseX=off  SenseY=off  SenseZ=off  SenseRad=off  SenseAzim=off  SenseDist=on  SenseInc=off  SenseXDot=off  SenseYDot=off  SenseZDot=off  SenseRadDot=off  SenseAzimDot=off  SenseDistDot=off  SenseIncDot=off  SenseXDDot=off  SenseYDDot=off  SenseZDDot=off  SenseRadDDot=off  SenseAzimDDot=off  SenseDistDDot=off  SenseIncDDot=off
  l0m : Constant  Value=Glenohumeral_l0(9)
  Scapula : PMIOPort  Side=Left
  Humerus : PMIOPort  Port=2  Side=Left
  Output : Outport
  Output1 : Outport  Port=2
  wires:
  PS-Simulink Converter/1 -> Output1/1, Active_factor_norm/1(lm), Passive_force_norm/1(lm)
  Passive_force_norm/1(Fp_norm) -> Sum/1
  Tlak->Tah/1 -> Output/1, Simulink-PS Converter/1
  Active_factor_norm/1(Fa_norm) -> Sum/2
  F0M/1 -> Tlak->Tah/1
  Sum/1 -> F0M/1
  Aktivace/1 -> Active_factor_norm/3(a)
  l0m/1 -> Active_factor_norm/2(l0), Passive_force_norm/2(l0)
  connections:
  PECM1_3/RConn1 -- Internal Force1/RConn1 -- Transform Sensor/RConn1
  PECM1_4/RConn1 -- Internal Force1/LConn1 -- Transform Sensor/LConn1
  Simulink-PS Converter/RConn1 -- Internal Force1/LConn2
  PECM1_4/LConn1 -- Scapula/RConn1
  Transform Sensor/RConn2 -- PS-Simulink Converter/LConn1
  PECM1_3/LConn1 -- Humerus/RConn1

== system run_2022/Glenohumeral/SUPSP ==
  Aktivace : Inport
  Active_factor_norm : MATLAB Function  TreatAsAtomicUnit=on
  F0M : Gain  Gain=Glenohumeral_F0M(10)
  Internal Force1 : sm_lib/Forces and Torques/Internal Force
  PECM1_3 : sm_lib/Frames and Transforms/Rigid Transform  TranslationMethod=Cartesian  TranslationStandardOffset=0  TranslationStandardOffsetUnits=m  TranslationStandardAxis=+Z  TranslationCartesianOffset=[0.04 0.031 0.006]  TranslationCartesianOffsetUnits=m  TranslationROffset=0  TranslationROffsetUnits=m  TranslationZOffset=0  TranslationZOffsetUnits=m  TranslationThetaOffset=0  TranslationThetaOffsetUnits=deg  RotationMethod=None  RotationAngleUnits=deg  RotationStandardAxis=+Z  RotationAngle=0.0  RotationArbitraryAxis=[0 0 1]  FollAlignAxisA=+X  BaseAlignAxisA=+Y  FollAlignAxisB=+Y  BaseAlignAxisB=+Z  RotationSequenceAxes=FollowerAxes  RotationSequence=XYX  RotationSequenceAngles=[0 0 0]  RotationSequenceAnglesUnits=deg  RotationMatrix=[1 0 0; 0 1 0; 0 0 1]  Quaternion=[1 0 0 0]
  PECM1_4 : sm_lib/Frames and Transforms/Rigid Transform  TranslationMethod=Cartesian  TranslationStandardOffset=0  TranslationStandardOffsetUnits=m  TranslationStandardAxis=+Z  TranslationCartesianOffset=[-0.056 -0.001 -0.041]  TranslationCartesianOffsetUnits=m  TranslationROffset=0  TranslationROffsetUnits=m  TranslationZOffset=0  TranslationZOffsetUnits=m  TranslationThetaOffset=0  TranslationThetaOffsetUnits=deg  RotationMethod=StandardAxis  RotationAngleUnits=deg  RotationStandardAxis=+Y  RotationAngle=90  RotationArbitraryAxis=[0 0 1]  FollAlignAxisA=+X  BaseAlignAxisA=+Y  FollAlignAxisB=+Y  BaseAlignAxisB=+Z  RotationSequenceAxes=FollowerAxes  RotationSequence=XYX  RotationSequenceAngles=[0 0 0]  RotationSequenceAnglesUnits=deg  RotationMatrix=[1 0 0; 0 1 0; 0 0 1]  Quaternion=[1 0 0 0]
  PS-Simulink Converter : nesl_utility/PS-Simulink Converter  PhysicalDomain=network_engine_domain  SubClassName=ps_output  LeftPortType=input  RightPortType=output  PseudoPeriodic=off  Frequencies=[]  VectorFormat=inherit  Unit=inherit  AffineConversion=off
  Passive_force_norm : MATLAB Function  TreatAsAtomicUnit=on
  Simulink-PS Converter : nesl_utility/Simulink-PS Converter  PhysicalDomain=network_engine_domain  SubClassName=ps_input  LeftPortType=input  RightPortType=output  PseudoPeriodic=off  Frequencies=[]  NoiseDistribution=none  NoiseParameters=[]  Unit=1  AffineConversion=off  FilteringAndDerivatives=provide  SimscapeFilterOrder=1  InputFilterTimeConstant=0.001  UdotUserProvided=0
  Sum : Sum  Inputs=|++
  Tlak->Tah : Gain  Gain=-1
  Transform Sensor : sm_lib/Frames and Transforms/Transform Sensor  MeasurementFrame=World  RotationSequence=XYX  SenseAngle=off  SenseAxis=off  SenseQ=off  SenseR=off  SenseRotationSequence=off  SenseOmegaX=off  SenseOmegaY=off  SenseOmegaZ=off  SenseQDot=off  SenseRDot=off  SenseRotationSequenceDot=off  SenseAlphaX=off  SenseAlphaY=off  SenseAlphaZ=off  SenseQDDot=off  SenseRDDot=off  SenseX=off  SenseY=off  SenseZ=off  SenseRad=off  SenseAzim=off  SenseDist=on  SenseInc=off  SenseXDot=off  SenseYDot=off  SenseZDot=off  SenseRadDot=off  SenseAzimDot=off  SenseDistDot=off  SenseIncDot=off  SenseXDDot=off  SenseYDDot=off  SenseZDDot=off  SenseRadDDot=off  SenseAzimDDot=off  SenseDistDDot=off  SenseIncDDot=off
  l0m : Constant  Value=Glenohumeral_l0(10)
  Scapula : PMIOPort  Side=Left
  Humerus : PMIOPort  Port=2  Side=Left
  Output : Outport
  Output1 : Outport  Port=2
  wires:
  Aktivace/1 -> Active_factor_norm/3(a)
  Sum/1 -> F0M/1
  F0M/1 -> Tlak->Tah/1
  Active_factor_norm/1(Fa_norm) -> Sum/2
  Passive_force_norm/1(Fp_norm) -> Sum/1
  l0m/1 -> Active_factor_norm/2(l0), Passive_force_norm/2(l0)
  Tlak->Tah/1 -> Output/1, Simulink-PS Converter/1
  PS-Simulink Converter/1 -> Output1/1, Active_factor_norm/1(lm), Passive_force_norm/1(lm)
  connections:
  PECM1_4/RConn1 -- Internal Force1/LConn1 -- Transform Sensor/LConn1
  PECM1_3/RConn1 -- Internal Force1/RConn1 -- Transform Sensor/RConn1
  PECM1_3/LConn1 -- Humerus/RConn1
  Transform Sensor/RConn2 -- PS-Simulink Converter/LConn1
  Simulink-PS Converter/RConn1 -- Internal Force1/LConn2
  PECM1_4/LConn1 -- Scapula/RConn1

== system run_2022/Glenohumeral/TMAJ ==
  Aktivace : Inport
  Active_factor_norm : MATLAB Function  TreatAsAtomicUnit=on
  F0M : Gain  Gain=Glenohumeral_F0M(11)
  Internal Force1 : sm_lib/Forces and Torques/Internal Force
  PECM1_3 : sm_lib/Frames and Transforms/Rigid Transform  TranslationMethod=Cartesian  TranslationStandardOffset=0  TranslationStandardOffsetUnits=m  TranslationStandardAxis=+Z  TranslationCartesianOffset=[0.004 -0.045 -0.007]  TranslationCartesianOffsetUnits=m  TranslationROffset=0  TranslationROffsetUnits=m  TranslationZOffset=0  TranslationZOffsetUnits=m  TranslationThetaOffset=0  TranslationThetaOffsetUnits=deg  RotationMethod=None  RotationAngleUnits=deg  RotationStandardAxis=+Z  RotationAngle=0.0  RotationArbitraryAxis=[0 0 1]  FollAlignAxisA=+X  BaseAlignAxisA=+Y  FollAlignAxisB=+Y  BaseAlignAxisB=+Z  RotationSequenceAxes=FollowerAxes  RotationSequence=XYX  RotationSequenceAngles=[0 0 0]  RotationSequenceAnglesUnits=deg  RotationMatrix=[1 0 0; 0 1 0; 0 0 1]  Quaternion=[1 0 0 0]
  PECM1_4 : sm_lib/Frames and Transforms/Rigid Transform  TranslationMethod=Cartesian  TranslationStandardOffset=0  TranslationStandardOffsetUnits=m  TranslationStandardAxis=+Z  TranslationCartesianOffset=[-0.045 -0.106 -0.002]  TranslationCartesianOffsetUnits=m  TranslationROffset=0  TranslationROffsetUnits=m  TranslationZOffset=0  TranslationZOffsetUnits=m  TranslationThetaOffset=0  TranslationThetaOffsetUnits=deg  RotationMethod=StandardAxis  RotationAngleUnits=deg  RotationStandardAxis=+Y  RotationAngle=90  RotationArbitraryAxis=[0 0 1]  FollAlignAxisA=+X  BaseAlignAxisA=+Y  FollAlignAxisB=+Y  BaseAlignAxisB=+Z  RotationSequenceAxes=FollowerAxes  RotationSequence=XYX  RotationSequenceAngles=[0 0 0]  RotationSequenceAnglesUnits=deg  RotationMatrix=[1 0 0; 0 1 0; 0 0 1]  Quaternion=[1 0 0 0]
  PS-Simulink Converter : nesl_utility/PS-Simulink Converter  PhysicalDomain=network_engine_domain  SubClassName=ps_output  LeftPortType=input  RightPortType=output  PseudoPeriodic=off  Frequencies=[]  VectorFormat=inherit  Unit=inherit  AffineConversion=off
  Passive_force_norm : MATLAB Function  TreatAsAtomicUnit=on
  Simulink-PS Converter : nesl_utility/Simulink-PS Converter  PhysicalDomain=network_engine_domain  SubClassName=ps_input  LeftPortType=input  RightPortType=output  PseudoPeriodic=off  Frequencies=[]  NoiseDistribution=none  NoiseParameters=[]  Unit=1  AffineConversion=off  FilteringAndDerivatives=provide  SimscapeFilterOrder=1  InputFilterTimeConstant=0.001  UdotUserProvided=0
  Sum : Sum  Inputs=|++
  Tlak->Tah : Gain  Gain=-1
  Transform Sensor : sm_lib/Frames and Transforms/Transform Sensor  MeasurementFrame=World  RotationSequence=XYX  SenseAngle=off  SenseAxis=off  SenseQ=off  SenseR=off  SenseRotationSequence=off  SenseOmegaX=off  SenseOmegaY=off  SenseOmegaZ=off  SenseQDot=off  SenseRDot=off  SenseRotationSequenceDot=off  SenseAlphaX=off  SenseAlphaY=off  SenseAlphaZ=off  SenseQDDot=off  SenseRDDot=off  SenseX=off  SenseY=off  SenseZ=off  SenseRad=off  SenseAzim=off  SenseDist=on  SenseInc=off  SenseXDot=off  SenseYDot=off  SenseZDot=off  SenseRadDot=off  SenseAzimDot=off  SenseDistDot=off  SenseIncDot=off  SenseXDDot=off  SenseYDDot=off  SenseZDDot=off  SenseRadDDot=off  SenseAzimDDot=off  SenseDistDDot=off  SenseIncDDot=off
  l0m : Constant  Value=Glenohumeral_l0(11)
  Scapula : PMIOPort  Side=Left
  Humerus : PMIOPort  Port=2  Side=Left
  Output : Outport
  Output1 : Outport  Port=2
  wires:
  l0m/1 -> Active_factor_norm/2(l0), Passive_force_norm/2(l0)
  Active_factor_norm/1(Fa_norm) -> Sum/2
  Sum/1 -> F0M/1
  Aktivace/1 -> Active_factor_norm/3(a)
  Passive_force_norm/1(Fp_norm) -> Sum/1
  Tlak->Tah/1 -> Output/1, Simulink-PS Converter/1
  F0M/1 -> Tlak->Tah/1
  PS-Simulink Converter/1 -> Output1/1, Active_factor_norm/1(lm), Passive_force_norm/1(lm)
  connections:
  PECM1_4/RConn1 -- Internal Force1/LConn1 -- Transform Sensor/LConn1
  PECM1_3/RConn1 -- Internal Force1/RConn1 -- Transform Sensor/RConn1
  PECM1_3/LConn1 -- Humerus/RConn1
  Simulink-PS Converter/RConn1 -- Internal Force1/LConn2
  Transform Sensor/RConn2 -- PS-Simulink Converter/LConn1
  PECM1_4/LConn1 -- Scapula/RConn1

== system run_2022/Glenohumeral/TMIN ==
  Aktivace : Inport
  Active_factor_norm : MATLAB Function  TreatAsAtomicUnit=on
  F0M : Gain  Gain=Glenohumeral_F0M(12)
  Internal Force1 : sm_lib/Forces and Torques/Internal Force
  PECM1_3 : sm_lib/Frames and Transforms/Rigid Transform  TranslationMethod=Cartesian  TranslationStandardOffset=0  TranslationStandardOffsetUnits=m  TranslationStandardAxis=+Z  TranslationCartesianOffset=[-0.008 -0.014 0.027]  TranslationCartesianOffsetUnits=m  TranslationROffset=0  TranslationROffsetUnits=m  TranslationZOffset=0  TranslationZOffsetUnits=m  TranslationThetaOffset=0  TranslationThetaOffsetUnits=deg  RotationMethod=None  RotationAngleUnits=deg  RotationStandardAxis=+Z  RotationAngle=0.0  RotationArbitraryAxis=[0 0 1]  FollAlignAxisA=+X  BaseAlignAxisA=+Y  FollAlignAxisB=+Y  BaseAlignAxisB=+Z  RotationSequenceAxes=FollowerAxes  RotationSequence=XYX  RotationSequenceAngles=[0 0 0]  RotationSequenceAnglesUnits=deg  RotationMatrix=[1 0 0; 0 1 0; 0 0 1]  Quaternion=[1 0 0 0]
  PECM1_4 : sm_lib/Frames and Transforms/Rigid Transform  TranslationMethod=Cartesian  TranslationStandardOffset=0  TranslationStandardOffsetUnits=m  TranslationStandardAxis=+Z  TranslationCartesianOffset=[-0.075 -0.053 -0.01]  TranslationCartesianOffsetUnits=m  TranslationROffset=0  TranslationROffsetUnits=m  TranslationZOffset=0  TranslationZOffsetUnits=m  TranslationThetaOffset=0  TranslationThetaOffsetUnits=deg  RotationMethod=StandardAxis  RotationAngleUnits=deg  RotationStandardAxis=+Y  RotationAngle=90  RotationArbitraryAxis=[0 0 1]  FollAlignAxisA=+X  BaseAlignAxisA=+Y  FollAlignAxisB=+Y  BaseAlignAxisB=+Z  RotationSequenceAxes=FollowerAxes  RotationSequence=XYX  RotationSequenceAngles=[0 0 0]  RotationSequenceAnglesUnits=deg  RotationMatrix=[1 0 0; 0 1 0; 0 0 1]  Quaternion=[1 0 0 0]
  PS-Simulink Converter : nesl_utility/PS-Simulink Converter  PhysicalDomain=network_engine_domain  SubClassName=ps_output  LeftPortType=input  RightPortType=output  PseudoPeriodic=off  Frequencies=[]  VectorFormat=inherit  Unit=inherit  AffineConversion=off
  Passive_force_norm : MATLAB Function  TreatAsAtomicUnit=on
  Simulink-PS Converter : nesl_utility/Simulink-PS Converter  PhysicalDomain=network_engine_domain  SubClassName=ps_input  LeftPortType=input  RightPortType=output  PseudoPeriodic=off  Frequencies=[]  NoiseDistribution=none  NoiseParameters=[]  Unit=1  AffineConversion=off  FilteringAndDerivatives=provide  SimscapeFilterOrder=1  InputFilterTimeConstant=0.001  UdotUserProvided=0
  Sum : Sum  Inputs=|++
  Tlak->Tah : Gain  Gain=-1
  Transform Sensor : sm_lib/Frames and Transforms/Transform Sensor  MeasurementFrame=World  RotationSequence=XYX  SenseAngle=off  SenseAxis=off  SenseQ=off  SenseR=off  SenseRotationSequence=off  SenseOmegaX=off  SenseOmegaY=off  SenseOmegaZ=off  SenseQDot=off  SenseRDot=off  SenseRotationSequenceDot=off  SenseAlphaX=off  SenseAlphaY=off  SenseAlphaZ=off  SenseQDDot=off  SenseRDDot=off  SenseX=off  SenseY=off  SenseZ=off  SenseRad=off  SenseAzim=off  SenseDist=on  SenseInc=off  SenseXDot=off  SenseYDot=off  SenseZDot=off  SenseRadDot=off  SenseAzimDot=off  SenseDistDot=off  SenseIncDot=off  SenseXDDot=off  SenseYDDot=off  SenseZDDot=off  SenseRadDDot=off  SenseAzimDDot=off  SenseDistDDot=off  SenseIncDDot=off
  l0m : Constant  Value=Glenohumeral_l0(12)
  Scapula : PMIOPort  Side=Left
  Humerus : PMIOPort  Port=2  Side=Left
  Output : Outport
  Output1 : Outport  Port=2
  wires:
  PS-Simulink Converter/1 -> Output1/1, Active_factor_norm/1(lm), Passive_force_norm/1(lm)
  F0M/1 -> Tlak->Tah/1
  l0m/1 -> Active_factor_norm/2(l0), Passive_force_norm/2(l0)
  Tlak->Tah/1 -> Output/1, Simulink-PS Converter/1
  Passive_force_norm/1(Fp_norm) -> Sum/1
  Aktivace/1 -> Active_factor_norm/3(a)
  Sum/1 -> F0M/1
  Active_factor_norm/1(Fa_norm) -> Sum/2
  connections:
  PECM1_4/RConn1 -- Internal Force1/LConn1 -- Transform Sensor/LConn1
  PECM1_3/RConn1 -- Internal Force1/RConn1 -- Transform Sensor/RConn1
  PECM1_4/LConn1 -- Scapula/RConn1
  PECM1_3/LConn1 -- Humerus/RConn1
  Transform Sensor/RConn2 -- PS-Simulink Converter/LConn1
  Simulink-PS Converter/RConn1 -- Internal Force1/LConn2
